simulink model "aero_radmod"  (Simulink 6.0)
settings: Solver=ode5  SolverMode=SingleTasking  StartTime=0.0  StopTime=100  FixedStep=0.1  MaxStep=0.1  RelTol=1e-3  AbsTol=1e-6
PreLoadFcn:
  | aero_raddat;
StopFcn:
  | aero_radplot;
values from neighbouring files (symbols this model uses):
  deltat = 1    [aero_raddat.m]
  g = 32.2    [aero_raddat.m]    (also in autopilot_data.mat; f14dat.m)
  Speed = 400    [aero_raddat.m]
  tauc = 5    [aero_raddat.m]
  tauT = 4    [aero_raddat.m]
libraries: simulink x2
CloseFcn:
  | h=findobj('type','figure');if ~isempty(h);close(h);end
settings Model: CovMetricSettings=d  Creator=The MathWorks Inc.  LastModifiedBy=batserve  ExtModeTrigMode=oneshot  ExtModeArmWhenConnect=off  ExtModeAutoUpdateStatusClock=off
settings DataIOCC: LimitDataPoints=off  SaveOutput=off  TimeSaveName=t_sim
settings OptimizationCC: BlockReduction=off  BooleanDataType=off
settings DebuggingCC: CheckExecutionContextPreStartOutputMsg=on  CheckExecutionContextRuntimeOutputMsg=on  SolverPrmCheckMsg=none
settings HardwareCC: TargetUnknown=on
settings RTWCC: MakeCommand="make_rtw  OPTS=-D"  TemplateMakefile=grt_vc.tmf

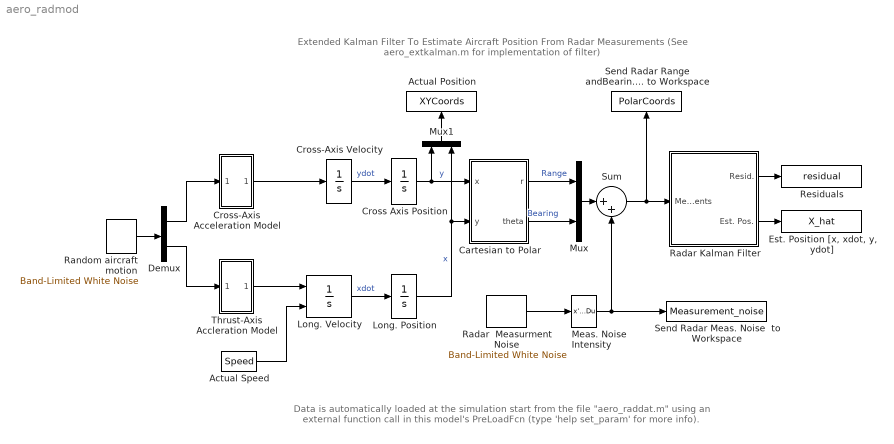
== system aero_radmod ==
  note: Data is automatically loaded at the simulation start from the file
      | "aero_raddat.m"
      | using an external function call in this model's PreLoadFcn
      | (type 'help set_param' for more info).
  note: Extended Kalman Filter To Estimate Aircraft Position From Radar Measurements
      | (See aero_extkalman.m for implementation of filter)
  Actual Position : ToWorkspace  VariableName=XYCoords  SaveFormat=Array
      settings: Orientation=up
  Actual Speed : Constant  Value=Speed
  Cartesian to Polar : Subsystem  PropExecContextAcrossSSBoundary=on
      mask Type: [x,y]->[r,theta]
      mask Description:
      | Tranformation from cartesian to polar
      | coordinates.
      | r=sqrt(x^2+y^2), theta=atan(y/x)
      mask Help: Unmask this block for more help.
      mask Display: plot(0,0,100,100,[24,20,15,20,20],[85,95,85,95,20],[80,20,95,85,95,85],[70,20,20,15,20,24],[56,56,55,52,50,46],[20,26,31,35,38,42])
  "Cross Axis Position " : Integrator
  Cross-Axis Acceleration Model : Subsystem  PropExecContextAcrossSSBoundary=on
  Cross-Axis Velocity : Integrator
  Demux : Demux  Outputs=2
  "Est. Position [x, xdot, y, ydot]" : ToWorkspace  VariableName=X_hat  SampleTime=-1  SaveFormat=Array
  Long. Position : Integrator
  Long. Velocity : Integrator  InitialConditionSource=external
  Meas. Noise Intensity : StateSpace  A=[]  B=[]  C=[]  D=K  mask(Matrix Gain){@1=[300 0; 0 .01]}
      mask prompts: @1 "Gain matrix:"
      mask help: Matrix Gain.
      mask init:
      | K = @1;
      mask Help: Multiplies input vector by entered matrix to produce output vector (y=Au).
      mask Display: disp('K')
  Mux : Mux  Inputs=2
  Mux1 : Mux  Orientation=up  Inputs=2
  Radar Kalman Filter : Subsystem  PropExecContextAcrossSSBoundary=on
  Radar  Measurment Noise : simulink/Sources/Band-Limited White Noise  Cov=[1 1]  Ts=0.1  seed=[52341 62341]
  Random aircraft motion : simulink/Sources/Band-Limited White Noise  Cov=[0.001 .001]  Ts=0.1  seed=[58413 74925]
  Residuals : ToWorkspace  VariableName=residual  SampleTime=-1  SaveFormat=Array
  Send Radar Meas. Noise  to Workspace : ToWorkspace  VariableName=Measurement_noise  SaveFormat=Array
  Send Radar Range andBearing  Angle Meas. to Workspace : ToWorkspace  VariableName=PolarCoords  SampleTime=-1  SaveFormat=Array
      settings: Orientation=up
  Sum : Sum  Inputs=|++  SaturateOnIntegerOverflow=on  InputSameDT=on
  Thrust-Axis Accleration Model : Subsystem  PropExecContextAcrossSSBoundary=on
  wires:
  Long. Position/1 -> Mux1/2, Cartesian to Polar/2(y)  "x"
  Cartesian to Polar/2(theta) -> Mux/2  "Bearing"
  Cartesian to Polar/1(r) -> Mux/1  "Range"
  Mux/1 -> Sum/1
  Sum/1 -> Radar Kalman Filter/1(Measurements), Send Radar Range andBearing  Angle Meas. to Workspace/1
  "Cross Axis Position "/1 -> Mux1/1, Cartesian to Polar/1(x)  "y"
  Cross-Axis Acceleration Model/1(out_1) -> Cross-Axis Velocity/1
  Cross-Axis Velocity/1 -> "Cross Axis Position "/1  "ydot"
  Actual Speed/1 -> Long. Velocity/2
  Long. Velocity/1 -> Long. Position/1  "xdot"
  Thrust-Axis Accleration Model/1(Accleration) -> Long. Velocity/1
  Radar Kalman Filter/1(Resid.) -> Residuals/1
  Demux/1 -> Cross-Axis Acceleration Model/1(Inport)
  Demux/2 -> Thrust-Axis Accleration Model/1(Force)
  Random aircraft motion/1 -> Demux/1
  Radar Kalman Filter/2(Est. Pos.) -> "Est. Position [x, xdot, y, ydot]"/1
  Mux1/1 -> Actual Position/1
  Radar  Measurment Noise/1 -> Meas. Noise Intensity/1
  Meas. Noise Intensity/1 -> Send Radar Meas. Noise  to Workspace/1, Sum/2

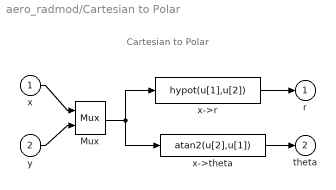
== system aero_radmod/Cartesian to Polar ==
  note: Cartesian to Polar
  x : Inport  Port=1  LatchInput=off
  y : Inport  Port=2  LatchInput=off
  Mux : Mux  Inputs=2
  x->r : Fcn  Expr=hypot(u[1],u[2])
  x->theta : Fcn  Expr=atan2(u[2],u[1])
  r : Outport  InitialOutput=0
  theta : Outport  Port=2  InitialOutput=0
  wires:
  Mux/1 -> x->r/1, x->theta/1
  x->r/1 -> r/1
  x/1 -> Mux/1
  y/1 -> Mux/2
  x->theta/1 -> theta/1

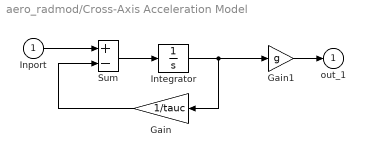
== system aero_radmod/Cross-Axis Acceleration Model ==
  Inport : Inport  Port=1  LatchInput=off
  Gain : Gain  Orientation=left  Gain=1/tauc  SaturateOnIntegerOverflow=on
  Gain1 : Gain  Gain=g  SaturateOnIntegerOverflow=on
  Integrator : Integrator
  Sum : Sum  Inputs=+-  SaturateOnIntegerOverflow=on  InputSameDT=on
  out_1 : Outport  InitialOutput=0
  wires:
  Inport/1 -> Sum/1
  Gain/1 -> Sum/2
  Integrator/1 -> Gain1/1, Gain/1
  Sum/1 -> Integrator/1
  Gain1/1 -> out_1/1

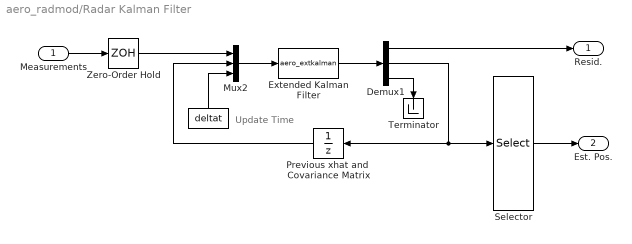
== system aero_radmod/Radar Kalman Filter ==
  note: Update Time
  Measurements : Inport  Port=1  LatchInput=off
  " " : Constant  Orientation=up  Value=deltat
  Demux1 : Demux  Outputs=[2 20 1]
  Extended Kalman Filter : MATLABFcn  MATLABFcn=aero_extkalman  OutputDimensions=23
  Mux2 : Mux  Inputs=3
  Previous xhat and  Covariance Matrix : UnitDelay  Orientation=left  X0=[0.001; 0.01; 0.001; 400; zeros(16,1)]  SampleTime=deltat
  Selector : Selector  Elements=[1:4]  InputPortWidth=20
  Terminator : Terminator
      settings: Orientation=down
  Zero-Order Hold : ZeroOrderHold  SampleTime=deltat
  Resid. : Outport  InitialOutput=0
  Est. Pos. : Outport  Port=2  InitialOutput=0
  wires:
  Measurements/1 -> Zero-Order Hold/1
  Extended Kalman Filter/1 -> Demux1/1
  Zero-Order Hold/1 -> Mux2/1
  Selector/1 -> Est. Pos./1
  Demux1/1 -> Resid./1
  Demux1/2 -> Previous xhat and  Covariance Matrix/1, Selector/1
  " "/1 -> Mux2/3
  Previous xhat and  Covariance Matrix/1 -> Mux2/2
  Mux2/1 -> Extended Kalman Filter/1
  Demux1/3 -> Terminator/1

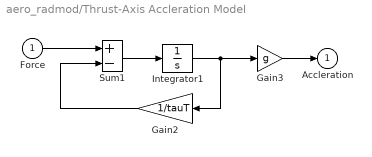
== system aero_radmod/Thrust-Axis Accleration Model ==
  Force : Inport  Port=1  LatchInput=off
  Gain2 : Gain  Orientation=left  Gain=1/tauT  SaturateOnIntegerOverflow=on
  Gain3 : Gain  Gain=g  SaturateOnIntegerOverflow=on
  Integrator1 : Integrator
  Sum1 : Sum  Inputs=+-  SaturateOnIntegerOverflow=on  InputSameDT=on
  Accleration : Outport  InitialOutput=0
  wires:
  Force/1 -> Sum1/1
  Gain2/1 -> Sum1/2
  Integrator1/1 -> Gain3/1, Gain2/1
  Sum1/1 -> Integrator1/1
  Gain3/1 -> Accleration/1
